simulink model "M11"  (R2021b)
settings: Solver=VariableStepAuto  StartTime=0.0  StopTime=10.0  RelTol=1e-3
values from neighbouring files (symbols this model uses):
  K1 = Wn^2    [M10.m]    (also in M11.m = wn^2)
  K2 = 2*zeta*Wn    [M10.m]    (also in M11.m = 2*zeta*wn - 1)
  wn = pi/(tp*sqrt(1-zeta^2))    [M11.m]
  zeta = rzeta(4)    [M10.m]    (also in M11.m = 1/sqrt(a^2 + 1))
settings Model: Creator=Student  LastModifiedBy=Student

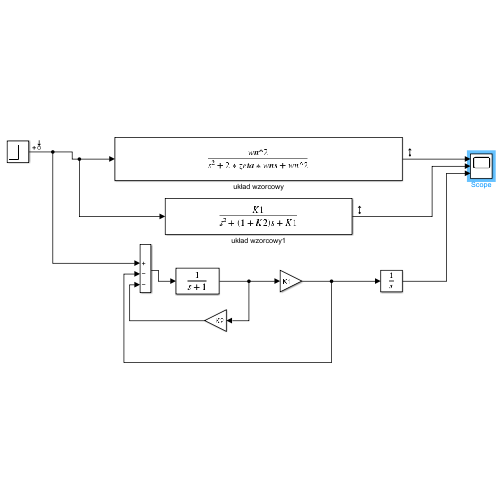
[thumbnail: Simulink's stored preview of the top-level diagram]
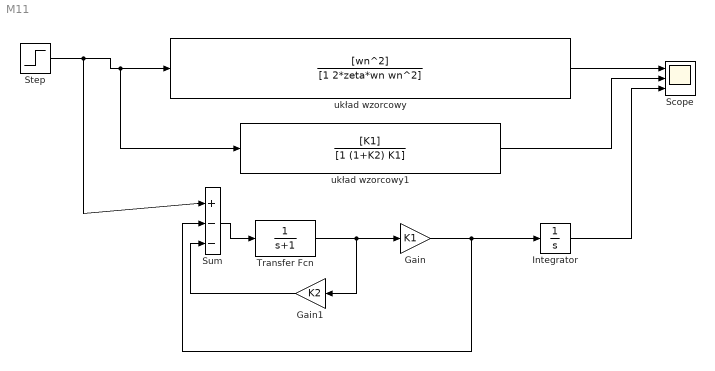
== system M11 ==
  Gain : Gain  Gain=K1
  Gain1 : Gain  Gain=K2
  Integrator : Integrator
  Scope : Scope  NumInputPorts=3
  Step : Step  SampleTime=0
  Sum : Sum  Inputs=|+--
  Transfer Fcn : TransferFcn  Denominator=[1 1]
  układ wzorcowy : TransferFcn  Numerator=[wn^2]  Denominator=[1 2*zeta*wn wn^2]
  układ wzorcowy1 : TransferFcn  Numerator=[K1]  Denominator=[1 (1+K2) K1]
  wires:
  układ wzorcowy/1 -> Scope/1
  Step/1 -> Sum/1, układ wzorcowy1/1, układ wzorcowy/1
  Gain1/1 -> Sum/3
  Sum/1 -> Transfer Fcn/1
  Transfer Fcn/1 -> Gain1/1, Gain/1
  Gain/1 -> Integrator/1, Sum/2
  układ wzorcowy1/1 -> Scope/2
  Integrator/1 -> Scope/3
